simulink model "Landing"  (R2019a)
settings: Solver=VariableStepAuto  StartTime=0.0  StopTime=120  RelTol=1e-3
values from neighbouring files (symbols this model uses):
  airport_elevation = 3000    [Ch7_Landing.m]    (also in Landing_Script.m)
  con_init = [0, 0, 0, 0, 0]'    [Ch7_Landing.m]    (also in Landing_Script.m)
  con_trim = [xu(3), xu(7), xu(8), xu(5), xu(11)]'    [Ch7_Landing.m]    (also in Landing_Script.m)
  init_x_pos = - ( time_to_intercept*con_trim(2)                     + (con_trim(1) - airport_elevation)                         / (tand(glideslope)) )    [Ch7_Landing.m]    (also in Landing_Script.m)
  SS_long = ss(A_long, B_long, C_long, D_long)    [Ch4_0_TrimLin.m]    (also in Ch7_Landing.m = FiveDoF.SS_long; Landing_Script.m = FiveDoF.SS_long; trim_lin.m = "")
  trim_elevator = xu(14)    [Ch7_Landing.m]    (also in Landing_Script.m)
  trim_thrust = xu(13)    [Ch7_Landing.m]    (also in Landing_Script.m)
undefined symbols (not defined in the file or in its folder): K_a, K_q
libraries: simulink_extras x4, simulink x2
settings Model: Creator=tblaha  LastModifiedBy=tblaha

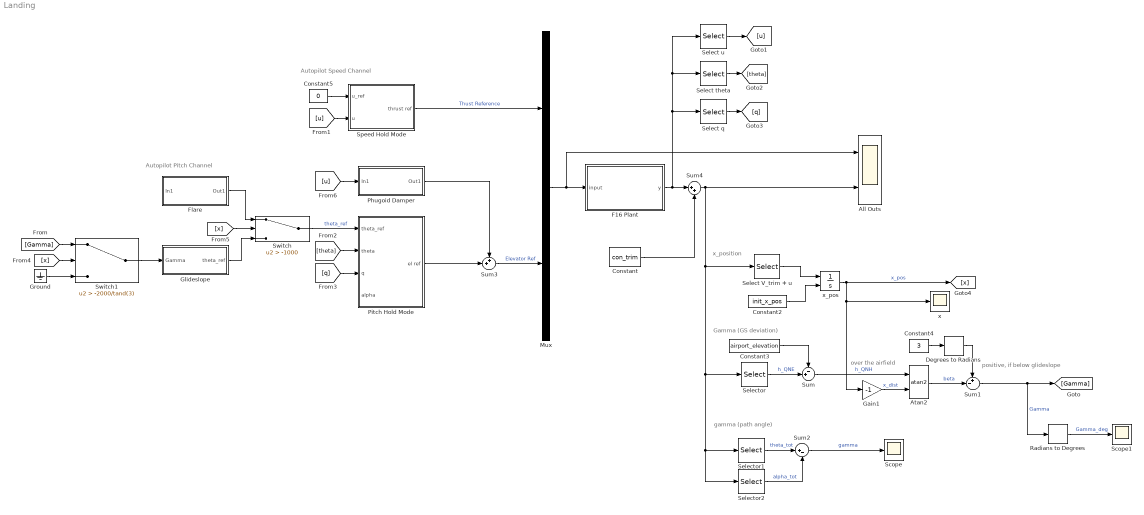
== system Landing ==
  note: Autopilot Speed Channel
  note: gamma (path angle)
  note: positive, if
      | below glideslope
  note: Gamma (GS deviation)
  note: over the airfield
  note: x_position
  note: Autopilot Pitch Channel
  All Outs : Scope  NumInputPorts=2
  Atan2 : Trigonometry  Operator=atan2
  Constant : Constant  Value=con_trim
  Constant2 : Constant  Value=init_x_pos
  Constant3 : Constant  Value=airport_elevation
  Constant4 : Constant  Value=3
  Constant5 : Constant  Value=0
  Degrees to Radians : simulink_extras/Transformations/Degrees to Radians
  F16 Plant : Subsystem
  Flare : Subsystem
  Gain1 : Gain  Gain=-1
  Glideslope : Subsystem
  Ground : Ground
  Mux : Mux  Inputs=2
  Phugoid Damper : Subsystem
  Pitch Hold Mode : Subsystem
  Radians to Degrees : simulink_extras/Transformations/Radians to Degrees
  Scope : Scope
  Scope1 : Scope
  Select V_trim + u : Selector  InputPortWidth=5  IndexOptions=Index vector (dialog)  Indices=[2]  OutputSizes=1
  Select q : Selector  InputPortWidth=5  IndexOptions=Index vector (dialog)  Indices=4  OutputSizes=1
  Select theta : Selector  InputPortWidth=5  IndexOptions=Index vector (dialog)  Indices=4  OutputSizes=1
  Select u : Selector  InputPortWidth=5  IndexOptions=Index vector (dialog)  Indices=[2]  OutputSizes=1
  Selector : Selector  InputPortWidth=5  IndexOptions=Index vector (dialog)  Indices=1  OutputSizes=1
  Selector1 : Selector  InputPortWidth=5  IndexOptions=Index vector (dialog)  Indices=4  OutputSizes=1
  Selector2 : Selector  InputPortWidth=5  IndexOptions=Index vector (dialog)  Indices=3  OutputSizes=1
  Speed Hold Mode : Subsystem
  Sum : Sum  Inputs=-+|
  Sum1 : Sum  Inputs=+-|
  Sum2 : Sum  Inputs=|+-
  Sum3 : Sum  Inputs=++|
  Sum4 : Sum  Inputs=|++
  Switch : Switch  Criteria=u2 > Threshold  Threshold=-1000
  Switch1 : Switch  Criteria=u2 > Threshold  Threshold=-2000/tand(3)
  x : Scope
  x_pos : Integrator  InitialConditionSource=external
  wires:
  Glideslope/1(theta_ref) -> Switch/3
  Flare/1(Out1) -> Switch/1
  Switch/1 -> Pitch Hold Mode/1(theta_ref)  "theta_ref"
  [x] -> Switch/2
  Constant2/1 -> x_pos/2
  Select V_trim + u/1 -> x_pos/1
  x_pos/1 -> Gain1/1, x/1, [x]  "x_pos"
  F16 Plant/1(y) -> Sum4/1, Select theta/1, Select u/1, Select q/1
  Pitch Hold Mode/1(el ref) -> Sum3/2
  Selector/1 -> Sum/2  "h_QNE"
  Constant3/1 -> Sum/1
  Sum/1 -> Atan2/1  "h_QNH"
  Gain1/1 -> Atan2/2  "x_dist"
  Atan2/1 -> Sum1/2  "beta"
  Constant4/1 -> Degrees to Radians/1
  Degrees to Radians/1 -> Sum1/1
  Sum1/1 -> Radians to Degrees/1, [Gamma]  "Gamma"
  Selector1/1 -> Sum2/1  "theta_tot"
  Selector2/1 -> Sum2/2  "alpha_tot"
  Sum2/1 -> Scope/1  "gamma"
  [Gamma] -> Switch1/1
  Speed Hold Mode/1(thrust ref) -> Mux/1  "Thust Reference"
  [theta] -> Pitch Hold Mode/2(theta)
  [q] -> Pitch Hold Mode/3(q)
  Constant5/1 -> Speed Hold Mode/1(u_ref)
  Select u/1 -> [u]
  [u] -> Speed Hold Mode/2(u)
  Select theta/1 -> [theta]
  Select q/1 -> [q]
  Mux/1 -> All Outs/1, F16 Plant/1(input)
  Radians to Degrees/1 -> Scope1/1  "Gamma_deg"
  [x] -> Switch1/2
  Ground/1 -> Switch1/3
  Switch1/1 -> Glideslope/1(Gamma)
  [u] -> Phugoid Damper/1(In1)
  Sum3/1 -> Mux/2  "Elevator Ref"
  Phugoid Damper/1(Out1) -> Sum3/1
  Constant/1 -> Sum4/2
  Sum4/1 -> All Outs/2, Select V_trim + u/1, Selector2/1, Selector1/1, Selector/1

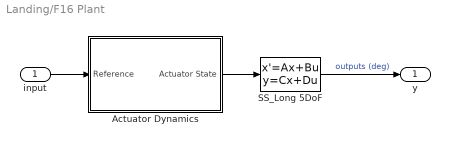
== system Landing/F16 Plant ==
  input : Inport
  Actuator Dynamics : Subsystem
  SS_Long 5DoF : StateSpace  A=SS_long.A  B=SS_long.B  C=SS_long.C  D=SS_long.D  InitialCondition=con_init
  y : Outport
  wires:
  input/1 -> Actuator Dynamics/1(Reference)
  SS_Long 5DoF/1 -> y/1  "outputs (deg)"
  Actuator Dynamics/1(Actuator State) -> SS_Long 5DoF/1

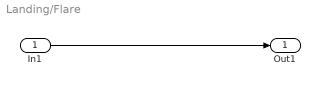
== system Landing/Flare ==
  In1 : Inport
  Out1 : Outport
  wires:
  In1/1 -> Out1/1

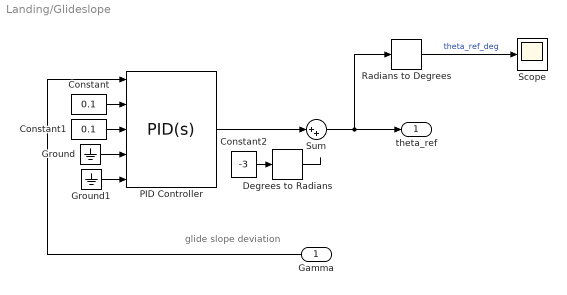
== system Landing/Glideslope ==
  note: glide slope deviation
  Gamma : Inport
  Constant : Constant  Value=0.1
  Constant1 : Constant  Value=0.1
  Constant2 : Constant  Value=-3
  Degrees to Radians : simulink_extras/Transformations/Degrees to Radians
  Ground : Ground
  Ground1 : Ground
  PID Controller : simulink/Continuous/PID Controller  Controller=PID  Form=Ideal  TimeDomain=Continuous-time  SampleTime=-1  IntegratorMethod=Forward Euler  FilterMethod=Forward Euler  ControllerParametersSource=external  P=1  I=0.1  D=0  UseFilter=on  N=100  TunerSelectOption=Transfer Function Based (PID Tuner App)  InitialConditionSource=internal  InitialConditionForIntegrator=0  InitialConditionForFilter=0  DifferentiatorICPrevScaledInput=0  ExternalReset=none  TrackingMode=off  Kt=1  LimitOutput=off  UpperSaturationLimit=inf  LowerSaturationLimit=-inf  LinearizeAsGain=on  AntiWindupMode=none  Kb=1  POutMin=[]  POutMax=[]  IOutMin=[]  IOutMax=[]  DOutMin=[]  DOutMax=[]  NOutMin=[]  NOutMax=[]  SumOutMin=[]  SumOutMax=[]  SaturationOutMin=[]  SaturationOutMax=[]  PParamMin=[]  PParamMax=[]  IParamMin=[]  IParamMax=[]  DParamMin=[]  DParamMax=[]  NParamMin=[]  NParamMax=[]  KbParamMin=[]  KbParamMax=[]  KtParamMin=[]  KtParamMax=[]  KbOutMin=[]  KbOutMax=[]  KtOutMin=[]  KtOutMax=[]  IntegratorOutMin=[]  IntegratorOutMax=[]  FilterOutMin=[]  FilterOutMax=[]  SumI1OutMin=[]  SumI1OutMax=[]  SumI2OutMin=[]  SumI2OutMax=[]  SumI3OutMin=[]  SumI3OutMax=[]  SumI4OutMin=[]  SumI4OutMax=[]  SumDOutMin=[]  SumDOutMax=[]  DifferentiatorOutMin=[]  DifferentiatorOutMax=[]  FilterDiffOutCoefMin=[]  FilterDiffOutCoefMax=[]  ReciprocalOutMin=[]  ReciprocalOutMax=[]  SumDenOutMin=[]  SumDenOutMax=[]  SumNumOutMin=[]  SumNumOutMax=[]  DivideOutMin=[]  DivideOutMax=[]  IntegratorContinuousStateAttributes=''  IntegratorStateMustResolveToSignalObject=off  IntegratorRTWStateStorageClass=Auto  FilterContinuousStateAttributes=''  FilterStateMustResolveToSignalObject=off  FilterRTWStateStorageClass=Auto  ParallelPVariant=Passthrough  IdealPVariant=ExternalParameters  IVariant=ExternalParameters  DVariant=ExternalParameters  IntegratorVariant=Continuous  SatVariant=Disabled  AWVariant=Passthrough  PCopyVariant=Disabled  TRVariant=Disabled  FdbkBlocksVariant=Forward  IdealPFdbkVariant=Disabled  SatFdbkVariant=Disabled  DerivativeFilterVariant=ContFilter  NVariant=ExternalParameters  NCopyVariant=Disabled  FilterICVariant=InternalICsFilter  IntegratorICVariant=InternalICs  ExternalResetVariant=Disabled  TRSumVariant=Passthrough  SumFdbkVariant=Disabled  SumVariant=Sum_PID
  Radians to Degrees : simulink_extras/Transformations/Radians to Degrees
  Scope : Scope
  Sum : Sum  Inputs=|++
  theta_ref : Outport
  wires:
  Gamma/1 -> PID Controller/1
  Sum/1 -> theta_ref/1, Radians to Degrees/1
  Constant/1 -> PID Controller/2
  Constant1/1 -> PID Controller/3
  Ground/1 -> PID Controller/4
  Ground1/1 -> PID Controller/5
  Radians to Degrees/1 -> Scope/1  "theta_ref_deg"
  PID Controller/1 -> Sum/1
  Degrees to Radians/1 -> ?
  Constant2/1 -> Degrees to Radians/1

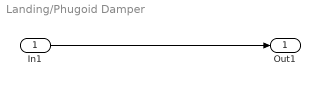
== system Landing/Phugoid Damper ==
  In1 : Inport
  Out1 : Outport
  wires:
  In1/1 -> Out1/1

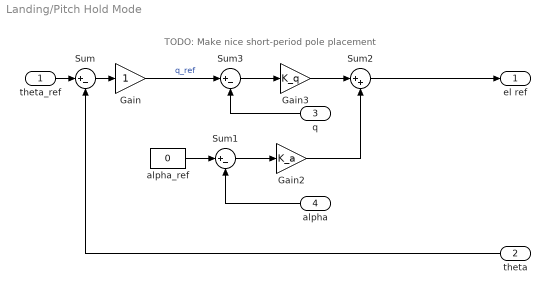
== system Landing/Pitch Hold Mode ==
  note: TODO: Make nice short-period pole placement
  theta_ref : Inport
  theta : Inport  Port=2
  q : Inport  Port=3
  alpha : Inport  Port=4
  Gain : Gain
  Gain2 : Gain  Gain=K_a
  Gain3 : Gain  Gain=K_q
  Sum : Sum  Inputs=|+-
  Sum1 : Sum  Inputs=|+-
  Sum2 : Sum  Inputs=|++
  Sum3 : Sum  Inputs=|+-
  alpha_ref : Constant  Value=0
  el ref : Outport
  wires:
  theta_ref/1 -> Sum/1
  Gain/1 -> Sum3/1  "q_ref"
  Sum/1 -> Gain/1
  theta/1 -> Sum/2
  Sum2/1 -> el ref/1
  alpha/1 -> Sum1/2
  alpha_ref/1 -> Sum1/1
  Sum1/1 -> Gain2/1
  Gain2/1 -> Sum2/2
  q/1 -> Sum3/2
  Sum3/1 -> Gain3/1
  Gain3/1 -> Sum2/1

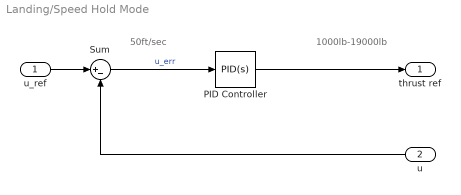
== system Landing/Speed Hold Mode ==
  note: 1000lb-19000lb
  note: 50ft/sec
  u_ref : Inport
  u : Inport  Port=2
  PID Controller : simulink/Continuous/PID Controller  Controller=PID  Form=Ideal  TimeDomain=Continuous-time  SampleTime=-1  IntegratorMethod=Forward Euler  FilterMethod=Forward Euler  ControllerParametersSource=internal  P=100  I=1  D=0  UseFilter=on  N=100  TunerSelectOption=Transfer Function Based (PID Tuner App)  InitialConditionSource=internal  InitialConditionForIntegrator=0  InitialConditionForFilter=0  DifferentiatorICPrevScaledInput=0  ExternalReset=none  TrackingMode=off  Kt=1  LimitOutput=off  UpperSaturationLimit=inf  LowerSaturationLimit=-inf  LinearizeAsGain=on  AntiWindupMode=none  Kb=1  POutMin=[]  POutMax=[]  IOutMin=[]  IOutMax=[]  DOutMin=[]  DOutMax=[]  NOutMin=[]  NOutMax=[]  SumOutMin=[]  SumOutMax=[]  SaturationOutMin=[]  SaturationOutMax=[]  PParamMin=[]  PParamMax=[]  IParamMin=[]  IParamMax=[]  DParamMin=[]  DParamMax=[]  NParamMin=[]  NParamMax=[]  KbParamMin=[]  KbParamMax=[]  KtParamMin=[]  KtParamMax=[]  KbOutMin=[]  KbOutMax=[]  KtOutMin=[]  KtOutMax=[]  IntegratorOutMin=[]  IntegratorOutMax=[]  FilterOutMin=[]  FilterOutMax=[]  SumI1OutMin=[]  SumI1OutMax=[]  SumI2OutMin=[]  SumI2OutMax=[]  SumI3OutMin=[]  SumI3OutMax=[]  SumI4OutMin=[]  SumI4OutMax=[]  SumDOutMin=[]  SumDOutMax=[]  DifferentiatorOutMin=[]  DifferentiatorOutMax=[]  FilterDiffOutCoefMin=[]  FilterDiffOutCoefMax=[]  ReciprocalOutMin=[]  ReciprocalOutMax=[]  SumDenOutMin=[]  SumDenOutMax=[]  SumNumOutMin=[]  SumNumOutMax=[]  DivideOutMin=[]  DivideOutMax=[]  IntegratorContinuousStateAttributes=''  IntegratorStateMustResolveToSignalObject=off  IntegratorRTWStateStorageClass=Auto  FilterContinuousStateAttributes=''  FilterStateMustResolveToSignalObject=off  FilterRTWStateStorageClass=Auto  ParallelPVariant=Passthrough  IdealPVariant=InternalParameters  IVariant=InternalParameters  DVariant=InternalParameters  IntegratorVariant=Continuous  SatVariant=Disabled  AWVariant=Passthrough  PCopyVariant=Disabled  TRVariant=Disabled  FdbkBlocksVariant=Forward  IdealPFdbkVariant=Disabled  SatFdbkVariant=Disabled  DerivativeFilterVariant=ContFilter  NVariant=InternalParameters  NCopyVariant=Disabled  FilterICVariant=InternalICsFilter  IntegratorICVariant=InternalICs  ExternalResetVariant=Disabled  TRSumVariant=Passthrough  SumFdbkVariant=Disabled  SumVariant=Sum_PID
  Sum : Sum  Inputs=|+-
  thrust ref : Outport
  wires:
  u_ref/1 -> Sum/1
  PID Controller/1 -> thrust ref/1
  Sum/1 -> PID Controller/1  "u_err"
  u/1 -> Sum/2

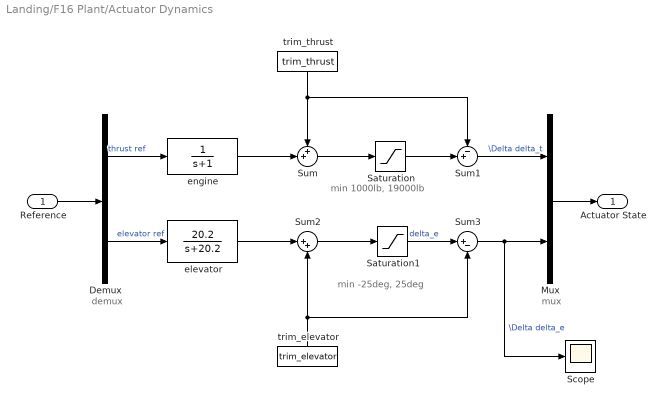
== system Landing/F16 Plant/Actuator Dynamics ==
  note: demux
  note: min 1000lb, 19000lb
  note: min -25deg, 25deg
  note: mux
  Reference : Inport
  Demux : Demux  Outputs=2
  Mux : Mux  Inputs=2
  Saturation : Saturate  UpperLimit=19000  LowerLimit=1000
  Saturation1 : Saturate  UpperLimit=25  LowerLimit=-25
  Scope : Scope
  Sum : Sum  Inputs=++|
  Sum1 : Sum  Inputs=-+|
  Sum2 : Sum  Inputs=|++
  Sum3 : Sum  Inputs=|+-
  elevator : TransferFcn  Numerator=[20.2]  Denominator=[1 20.2]
  engine : TransferFcn  Denominator=[1 1]
  trim_elevator : Constant  Value=trim_elevator
  trim_thrust : Constant  Value=trim_thrust
  Actuator State : Outport
  wires:
  Reference/1 -> Demux/1
  Demux/1 -> engine/1  "thrust ref"
  Demux/2 -> elevator/1  "elevator ref"
  engine/1 -> Sum/2
  Saturation/1 -> Sum1/2
  elevator/1 -> Sum2/1
  Saturation1/1 -> Sum3/1  "delta_e"
  Mux/1 -> Actuator State/1
  Sum/1 -> Saturation/1
  Sum1/1 -> Mux/1  "\\Delta delta_t"
  trim_thrust/1 -> Sum1/1, Sum/1
  Sum2/1 -> Saturation1/1
  Sum3/1 -> Scope/1, Mux/2  "\\Delta delta_e"
  trim_elevator/1 -> Sum3/2, Sum2/2
